simulink model "Rossler"  (Simulink 10.0)
settings: Solver=VariableStepAuto  StartTime=0.0  StopTime=8000  RelTol=1e-3
settings Model: Creator=szymo  LastModifiedBy=szymo
settings DataIOCC: SaveFormat=Dataset  ReturnWorkspaceOutputs=on
settings OptimizationCC: LifeSpan=auto
settings DebuggingCC: UnderspecifiedInitializationDetection=Simplified  MergeDetectMultiDrivingBlocksExec=error  SFUnexpectedBacktrackingDiag=error  SFNoUnconditionalDefaultTransitionDiag=error  SFExecutionAtInitializationDiag=warning  ArithmeticOperatorsInVariantConditions=error
settings HardwareCC: ProdBitPerPointer=64  ProdBitPerSizeT=64  ProdBitPerPtrDiffT=64  ProdLargestAtomicFloat=Float  ProdIntDivRoundTo=Zero  ProdEndianess=LittleEndian  ProdWordSize=64  ProdHWDeviceType=Intel->x86-64 (Windows64)
settings ModelReferenceCC: PropagateSignalLabelsOutOfModel=on
settings SFSimCC: SimUseLocalCustomCode=on  CustomCodeUndefinedFunction=FilterOut
settings RTWCC: RTWUseLocalCustomCode=on
settings CodeAppCC: StateflowObjectComments=off
settings GRTTargetCC: TargetLangStandard=C99 (ISO)  CombineOutputUpdateFcns=on  GRTInterface=off
settings ConfigComp: CovMetricSettings=dwe  CovHtmlReporting=off  CovSaveCumulativeToWorkspaceVar=off  CovSaveSingleToWorkspaceVar=off

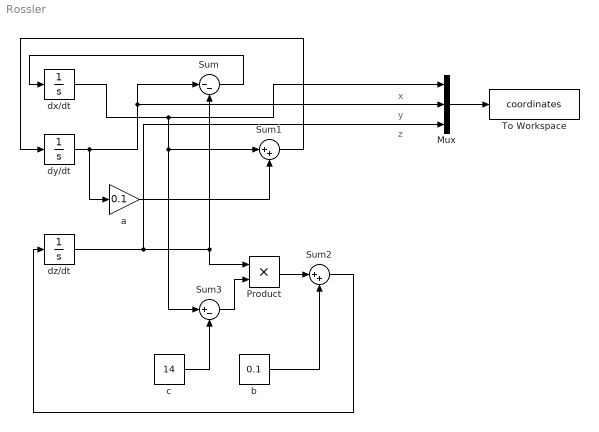
== system Rossler ==
  note: x
  note: z
  note: y
  Mux : Mux  Inputs=3
  Product : Product
  Sum : Sum  Inputs=|--
  Sum1 : Sum  Inputs=|++
  Sum2 : Sum  Inputs=|++
  Sum3 : Sum  Inputs=|+-
  To Workspace : ToWorkspace  VariableName=coordinates  SampleTime=-1
      settings: Save2DSignal=2-D array (concatenate along first dimension)
  a : Gain  Gain=0.1
  b : Constant  Value=0.1
  c : Constant  Value=14
  dx/dt : Integrator
  dy/dt : Integrator
  dz/dt : Integrator
  wires:
  Sum/1 -> dx/dt/1
  dy/dt/1 -> a/1, Mux/2, Sum/1
  dz/dt/1 -> Mux/3, Product/1, Sum/2
  dx/dt/1 -> Mux/1, Sum1/1, Sum3/1
  a/1 -> Sum1/2
  Sum1/1 -> dy/dt/1
  Product/1 -> Sum2/1
  b/1 -> Sum2/2
  c/1 -> Sum3/2
  Sum3/1 -> Product/2
  Sum2/1 -> dz/dt/1
  Mux/1 -> To Workspace/1
